simulink model "deska_ratunku"  (R2016a)
settings: Solver=VariableStepAuto  StartTime=0.0  StopTime=5000  RelTol=1e-3
values from neighbouring files (symbols this model uses):
  B = 0.0064    [Unit_3.m]    (also in reactor_pocz.m; unit_1.m; unit_4.m)
  C_lp_sg = 4314    [unit_4.m]
  c_p_PC = 5355    [Unit_3.m]    (also in unit_1.m = 5415)
  C_p_pc = 5197.6    [unit_4.m]
  c_p_PR = 6873.1    [Unit_3.m]    (also in unit_1.m)
  c_phi_1 = 2.98    [Unit_3.m]    (also in unit_1.m)
  c_phi_2 = -0.008448    [Unit_3.m]    (also in unit_1.m)
  C_psi = 13.75 * (10 ^ 6)    (= 13750000)    [Unit_3.m]    (also in reactor_pocz.m; unit_1.m; unit_4.m)
  C_vp_sg = 3449.8    [unit_4.m]
  cl_p_SG = 3809.9    [Unit_3.m]    (also in unit_1.m = 3871.3)
  cv_p_SG = 3635.6    [Unit_3.m]    (also in unit_1.m = 3489)
  E_evap_SG = 1.658 * (10 ^ 6)    (= 1658000)    [Unit_3.m]    (also in unit_1.m)
  E_evap_sg = 1.658 * (10 ^ 6)    (= 1658000)    [unit_4.m]
  K_T_SG = 9.5296 * (10 ^ 6)    (= 9529600)    [Unit_3.m]    (also in unit_1.m = 8400400)
  Kt_sg = 9.5296*(10^6)    (= 9529600)    [Unit_3.m]    (also in unit_4.m = 7554000)
  LAMBDA = 10 ^ -5    (= 1e-05)    [Unit_3.m]    (also in reactor_pocz.m; unit_1.m; unit_4.m)
  lambda = 0.1    [Unit_3.m]    (also in reactor_pocz.m; unit_1.m; unit_4.m)
  m_in = 1.4222    [Unit_3.m]    (also in unit_1.m)
  M_in = 2.19444    [unit_4.m]
  m_out = 2.11    [Unit_3.m]    (also in unit_1.m = 2.9722)
  M_out = 2.29722    [unit_4.m]
  M_PR = M_pc-V0_PC * (581.2 + 2.98*T_PC - 0.0848*(T_PC^2))    (= 1478515.60171)    [Unit_3.m]    (also in unit_1.m = 1445179.13836)
  m_SG = 119.31    [Unit_3.m]    (also in unit_1.m = 120.56)
  M_SG = 34920    [Unit_3.m]    (also in unit_1.m = 35611)
  P_1 = -1.223 * (10 ^ -4)    (= -0.0001223)    [Unit_3.m]    (also in reactor_pocz.m; unit_1.m = -0.0001322; unit_4.m = -0.0001286)
  P_2 = -5.502 * (10 ^ -5)    (= -5.502e-05)    [Unit_3.m]    (also in reactor_pocz.m; unit_1.m = -6.08e-05; unit_4.m = -6.79e-05)
  P_3 = -1.953 * (10 ^ -4)    (= -0.0001953)    [Unit_3.m]    (also in reactor_pocz.m; unit_1.m = -0.000285; unit_4.m = -0.0002887)
  S = 1938.9    [Unit_3.m]    (also in reactor_pocz.m; unit_1.m = 2859; unit_4.m = 2910.3)
  T_pc_hl = 295.21    [unit_4.m]
  T_PC_I = 258.85    [Unit_3.m]    (also in unit_1.m = 246.1)
  T_pc_i = 258.23    [unit_4.m]
  T_SG = 257.78    [Unit_3.m]    (also in unit_1.m = 255.13)
  T_SG_SW = 220.85    [Unit_3.m]    (also in unit_1.m = 219.65)
  T_sg_sw = 220.85    [unit_4.m]
  V0_PC = 242    [Unit_3.m]    (also in unit_1.m)
  V_0_pc = 242    [unit_4.m]
  W_loss_pc = 3.2733 * (10 ^ 8)    (= 327330000)    [unit_4.m]
  W_loss_PC = 2.996 * (10 ^ 7)    (= 29960000)    [Unit_3.m]    (also in unit_1.m = 224690000)
  W_loss_PR = 1.6823 * (10 ^ 5)    (= 168230)    [Unit_3.m]    (also in unit_1.m)
  W_loss_SG = 1.8932  * (10 ^ 7)    (= 18932000)    [Unit_3.m]    (also in unit_1.m = 191660)
  W_loss_sg = 1.324  * (10 ^ 7)    (= 13240000)    [unit_4.m]
libraries: simulink x2
settings Model: Creator=Użytkownik  LastModifiedBy=Użytkownik
settings GRTTargetCC: GeneratePreprocessorConditionals=Use local settings

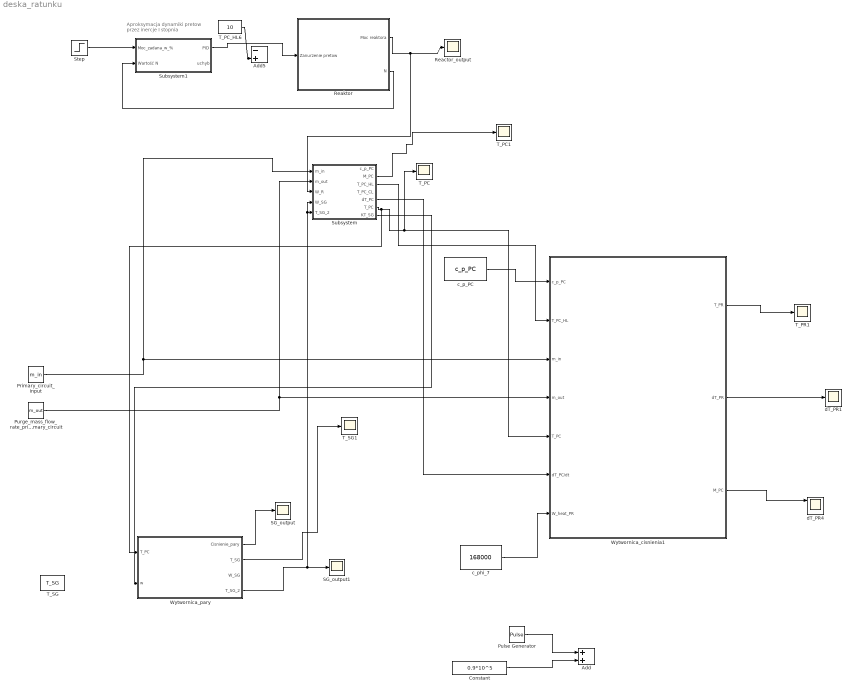
== system deska_ratunku ==
  note: Aproksymacja dynamiki
      | pretow przez inercje I stopnia
  Add : Sum
  Add5 : Sum  Inputs=-+
  Constant : Constant  Value=0.9*10^5
  Primary_circuit_input : Constant  Value=m_in
  Pulse Generator : DiscretePulseGenerator  PulseType=Time based  Amplitude=0.98*10^5  Period=6480  PulseWidth=80
  "Purge_mass_flow_rate_primary_circuit " : Constant  Value=m_out
  Reactor_output : Scope
  Reaktor : Subsystem
  SG_output : Scope
  SG_output1 : Scope
  Step : Step  Time=500  After=0.025  SampleTime=0
  Subsystem : Subsystem
  Subsystem1 : Subsystem
  T_PC : Scope
  T_PC1 : Scope
  T_PC_HL6 : Constant  Value=10
  T_PR1 : Scope
  T_SG : Constant  Value=T_SG
  T_SG1 : Scope
  Wytwornica_cisnienia1 : Subsystem
  Wytwornica_pary : Subsystem
  c_p_PC : Constant  Value=c_p_PC
  c_phi_7 : Constant  Value=168000
  dT_PR1 : Scope
  dT_PR4 : Scope  NumInputPorts=3
  wires:
  Reaktor/1(Moc reaktora) -> Subsystem/3(W_R), Reactor_output/1
  Wytwornica_pary/2(T_SG) -> T_SG1/1
  Primary_circuit_input/1 -> Subsystem/1(m_in), Wytwornica_cisnienia1/3(m_in)
  "Purge_mass_flow_rate_primary_circuit "/1 -> Subsystem/2(m_out), Wytwornica_cisnienia1/4(m_out)
  c_p_PC/1 -> Wytwornica_cisnienia1/1(c_p_PC)
  Subsystem/3(T_PC_HL) -> Wytwornica_cisnienia1/2(T_PC_HL)
  Wytwornica_cisnienia1/1(T_PR) -> T_PR1/1
  Wytwornica_cisnienia1/2(dT_PR) -> dT_PR1/1
  Pulse Generator/1 -> Add/1
  Constant/1 -> Add/2
  Subsystem/6(T_PC) -> Wytwornica_pary/1(T_PC), Wytwornica_cisnienia1/5(T_PC), T_PC/1
  Wytwornica_cisnienia1/3("M_PC ") -> dT_PR4/1
  c_phi_7/1 -> Wytwornica_cisnienia1/7(W_heat_PR)
  Subsystem/5(dT_PC) -> Wytwornica_cisnienia1/6(dT_PC/dt)
  Wytwornica_pary/1(Cisnienie_pary) -> SG_output/1
  Step/1 -> Subsystem1/1(Moc_zadana_w_%)
  Reaktor/2(N) -> Subsystem1/2(Wartość N)
  T_PC_HL6/1 -> Add5/2
  Subsystem/2(M_PC) -> T_PC1/1
  Subsystem1/1("PID ") -> Reaktor/1(Zanurzenie pretow)
  Subsystem/7("KT_SG ") -> Wytwornica_pary/2("w ")
  Wytwornica_pary/4(T_SG_2) -> Subsystem/4(W_SG), Subsystem/5(T_SG_2), SG_output1/1

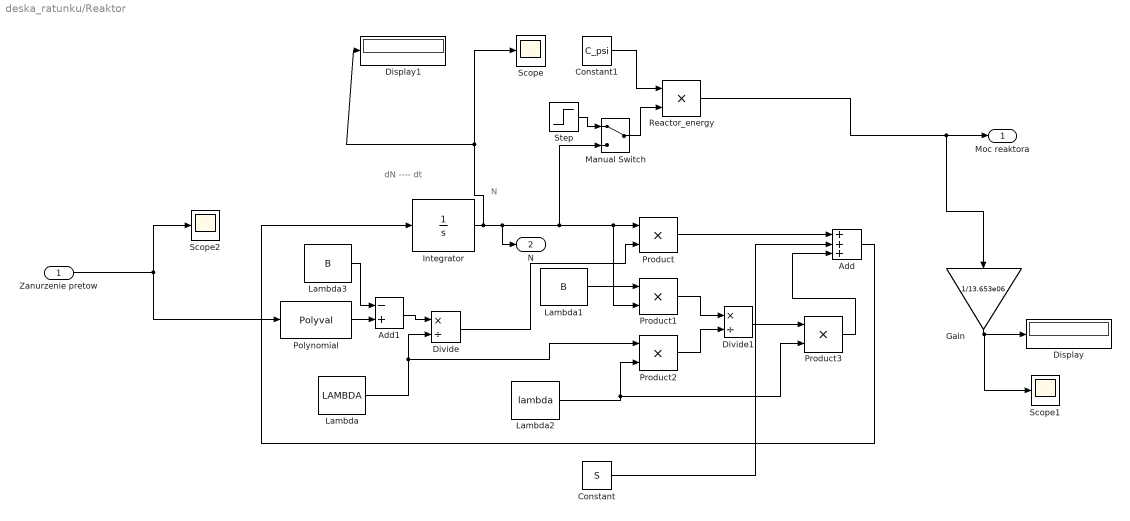
== system deska_ratunku/Reaktor ==
  note: N
  note: dN
      | ----
      | dt
  Zanurzenie pretow : Inport
  Add : Sum  Inputs=+++
  Add1 : Sum  Inputs=-+
  Constant : Constant  Value=S
  Constant1 : Constant  Value=C_psi
  Display : Display
  Display1 : Display
  Divide : Product  Inputs=*/
  Divide1 : Product  Inputs=*/
  Gain : Gain  Gain=1/13.653e06
  Integrator : Integrator  InitialCondition=99.3
  Lambda : Constant  Value=LAMBDA
  Lambda1 : Constant  Value=B
  Lambda2 : Constant  Value=lambda
  Lambda3 : Constant  Value=B
  Manual Switch : ManualSwitch
  Polynomial : Polyval  Coefs=[P_1, P_2, P_3]
  Product{,1..3} (4 alike) : Product
  Reactor_energy : Product
  Scope : Scope
  Scope1 : Scope
  Scope2 : Scope
  Step : Step  Time=500  Before=100.3  After=100.2  SampleTime=0
  Moc reaktora : Outport
  N : Outport  Port=2
  wires:
  Integrator/1 -> N/1, Manual Switch/2, Product1/2, Product/1, Display1/1, Scope/1
  Product/1 -> Add/1
  Constant/1 -> Add/2
  Add/1 -> Integrator/1
  Lambda/1 -> Product2/1, Divide/2
  Divide/1 -> Product/2
  Constant1/1 -> Reactor_energy/1
  Reactor_energy/1 -> Gain/1, Moc reaktora/1
  Lambda1/1 -> Product1/1
  Lambda2/1 -> Product2/2, Product3/2
  Product1/1 -> Divide1/1
  Product2/1 -> Divide1/2
  Divide1/1 -> Product3/1
  Product3/1 -> Add/3
  Lambda3/1 -> Add1/1
  Polynomial/1 -> Add1/2
  Add1/1 -> Divide/1
  Gain/1 -> Scope1/1, Display/1
  Zanurzenie pretow/1 -> Scope2/1, Polynomial/1
  Manual Switch/1 -> Reactor_energy/2
  Step/1 -> Manual Switch/1

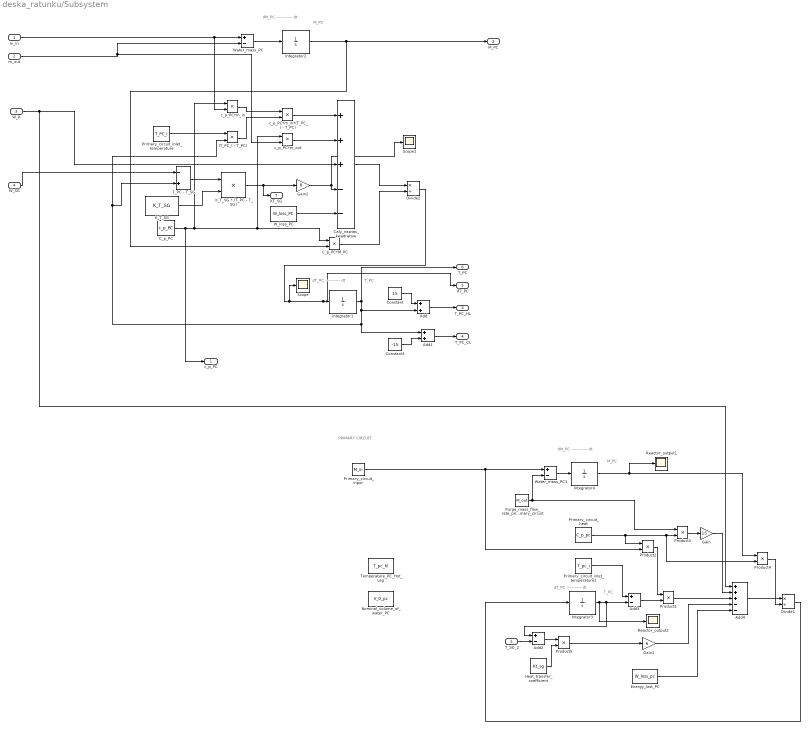
== system deska_ratunku/Subsystem ==
  note: dM_PC
      | ------------
      |      dt
  note: M_PC
  note: dT_PC
      | -----------
      |     dt
  note: T_PC
  note: dM_PC
      | ------------
      |      dt
  note: M_PC
  note: dT_PC
      | -----------
      |     dt
  note: T_PC
  note: PRIMARY CIRCUIT
  m_in : Inport
  m_out : Inport  Port=2
  W_R : Inport  Port=3
  W_SG : Inport  Port=4
  T_SG_2 : Inport  Port=5
  (T_PC_I - T_PC) : Product
  Add : Sum
  Add1 : Sum
  Add2 : Sum  Inputs=+-
  Add3 : Sum  Inputs=+-
  Add4 : Sum  Inputs=+++--
  C_p_PC : Constant  Value=c_p_PC
  C_p_PC*M_PC : Product
  Caly_nawias_kwadratow : Sum  Inputs=+++--
  Constant : Constant  Value=15
  Constant1 : Constant  Value=-15
  Divide1 : Product  Inputs=*/
  Divide2 : Product  Inputs=*/
  Energy_lost_PC : Constant  Value=W_loss_pc
  Gain : Gain  Gain=15
  Gain1 : Gain  Gain=6
  Gain2 : Gain  Gain=6
  Heat_transfer_coefficient : Constant  Value=Kt_sg
  Integrator1 : Integrator  InitialCondition=281.13
  Integrator2 : Integrator  InitialCondition=200000
  Integrator3 : Integrator  InitialCondition=281.13
  Integrator4 : Integrator  InitialCondition=200000
  K_T_SG : Constant  Value=K_T_SG
  K_T_SG * (T_PC - T_SG) : Product
  Nominal_volume_of_water_PC : Constant  Value=V_0_pc
  Primary_circuit_heat : Constant  Value=C_p_pc
  Primary_circuit_inlet_temperature : Constant  Value=T_PC_I
  Primary_circuit_inlet_temperature1 : Constant  Value=T_pc_i
  Primary_circuit_input : Constant  Value=M_in
  Product{1..5} (5 alike) : Product
  "Purge_mass_flow_rate_primary_circuit " : Constant  Value=M_out
  Reactor_output1 : Scope
  Reactor_output2 : Scope
  Scope : Scope
  Scope1 : Scope
  T_PC - T_SG : Sum  Inputs=-+
  Temperature_PC_Hot_Leg : Constant  Value=T_pc_hl
  W_loss_PC : Constant  Value=W_loss_PC
  Water_mass_PC : Sum  Inputs=+-
  Water_mass_PC1 : Sum  Inputs=+-
  c_p_PC*m_in : Product
  c_p_PC*m_in*(T_PC_I - T_PC) : Product
  c_p_PC*m_out : Product
  c_p_PC : Outport
  M_PC : Outport  Port=2
  T_PC_HL : Outport  Port=3
  T_PC_CL : Outport  Port=4
  dT_PC : Outport  Port=5
  T_PC : Outport  Port=6
  "KT_SG " : Outport  Port=7
  wires:
  m_in/1 -> c_p_PC*m_in/2, Water_mass_PC/1
  Water_mass_PC/1 -> Integrator2/1
  Integrator2/1 -> C_p_PC*M_PC/2, M_PC/1
  C_p_PC/1 -> c_p_PC/1, C_p_PC*M_PC/1, c_p_PC*m_out/1, c_p_PC*m_in/1
  C_p_PC*M_PC/1 -> Divide2/2
  Divide2/1 -> Scope/1, dT_PC/1, Integrator1/1
  Caly_nawias_kwadratow/1 -> Divide2/1
  c_p_PC*m_in*(T_PC_I - T_PC)/1 -> Caly_nawias_kwadratow/1
  c_p_PC*m_in/1 -> c_p_PC*m_in*(T_PC_I - T_PC)/1
  (T_PC_I - T_PC)/1 -> c_p_PC*m_in*(T_PC_I - T_PC)/2
  Primary_circuit_inlet_temperature/1 -> (T_PC_I - T_PC)/1
  c_p_PC*m_out/1 -> Caly_nawias_kwadratow/2
  W_loss_PC/1 -> Caly_nawias_kwadratow/5
  Constant/1 -> Add/1
  Constant1/1 -> Add1/2
  Integrator1/1 -> T_PC - T_SG/2, (T_PC_I - T_PC)/2, Add1/1, Add/2, T_PC/1
  Add1/1 -> T_PC_CL/1
  Add/1 -> T_PC_HL/1
  m_out/1 -> c_p_PC*m_out/2, Water_mass_PC/2
  Gain2/1 -> Caly_nawias_kwadratow/4, Scope1/1
  T_PC - T_SG/1 -> K_T_SG * (T_PC - T_SG)/1
  K_T_SG/1 -> K_T_SG * (T_PC - T_SG)/2
  K_T_SG * (T_PC - T_SG)/1 -> "KT_SG "/1, Gain2/1
  W_SG/1 -> T_PC - T_SG/1
  W_R/1 -> Add4/1, Caly_nawias_kwadratow/3
  Primary_circuit_input/1 -> Water_mass_PC1/1, Product2/2
  "Purge_mass_flow_rate_primary_circuit "/1 -> Water_mass_PC1/2, Product3/1
  Water_mass_PC1/1 -> Integrator4/1
  Integrator3/1 -> Reactor_output2/1, Add2/1, Add3/2
  Primary_circuit_inlet_temperature1/1 -> Add3/1
  Add3/1 -> Product1/2
  Product2/1 -> Product1/1
  Primary_circuit_heat/1 -> Product2/1, Product4/2, Product3/2
  Product1/1 -> Add4/3
  Product3/1 -> Gain/1
  Gain/1 -> Add4/2
  Product5/1 -> Gain1/1
  Gain1/1 -> Add4/4
  Add4/1 -> Divide1/1
  Integrator4/1 -> Reactor_output1/1, Product4/1
  Product4/1 -> Divide1/2
  Divide1/1 -> Integrator3/1
  Heat_transfer_coefficient/1 -> Product5/2
  Add2/1 -> Product5/1
  Energy_lost_PC/1 -> Add4/5
  T_SG_2/1 -> Add2/2

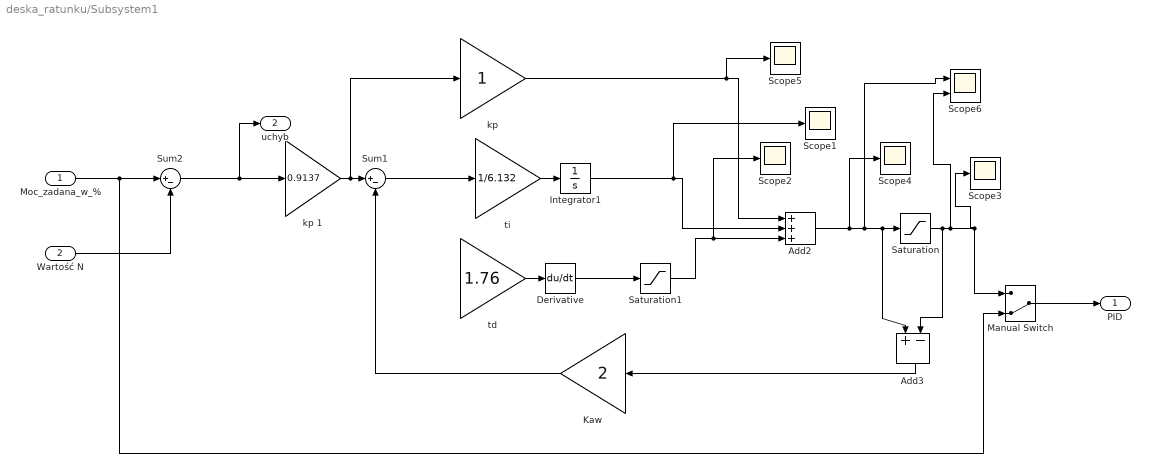
== system deska_ratunku/Subsystem1 ==
  Moc_zadana_w_% : Inport
  Wartość N : Inport  Port=2
  " kp " : Gain
  " kp 1" : Gain  Gain=0.9137
  Add2 : Sum  Inputs=+++
  Add3 : Sum  Inputs=+-
  Derivative : Derivative
  Integrator1 : Integrator
  "Kaw " : Gain  Gain=2
  Manual Switch : ManualSwitch  CurrentSetting=0
  Saturation : Saturate  UpperLimit=10  LowerLimit=0
  Saturation1 : Saturate  UpperLimit=10  LowerLimit=-10
  Scope{1..5} (5 alike) : Scope
  Scope6 : Scope  NumInputPorts=2
  Sum1 : Sum  Inputs=|+-
  Sum2 : Sum  Inputs=|+-
  "td " : Gain  Gain=1.76
  ti : Gain  Gain=1/6.132
  "PID " : Outport
  uchyb : Outport  Port=2
  wires:
  Derivative/1 -> Saturation1/1
  Add2/1 -> Scope6/1, Add3/1, Saturation/1, Scope4/1
  Saturation/1 -> Add3/2, Scope6/2, Scope3/1, Manual Switch/1
  Wartość N/1 -> Sum2/2
  Manual Switch/1 -> "PID "/1
  Moc_zadana_w_%/1 -> Manual Switch/2, Sum2/1
  ti/1 -> Integrator1/1
  "td "/1 -> Derivative/1
  Add3/1 -> "Kaw "/1
  " kp 1"/1 -> " kp "/1, Sum1/1
  Sum1/1 -> ti/1
  Saturation1/1 -> Scope2/1, Add2/3
  Integrator1/1 -> Scope1/1, Add2/2
  " kp "/1 -> Scope5/1, Add2/1
  Sum2/1 -> uchyb/1, " kp 1"/1
  "Kaw "/1 -> Sum1/2

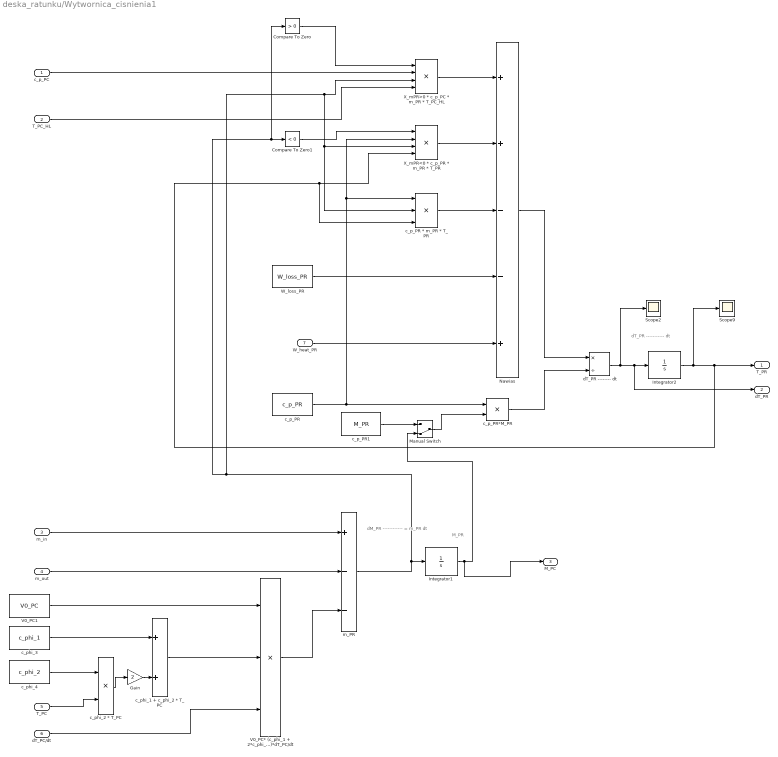
== system deska_ratunku/Wytwornica_cisnienia1 ==
  note: dT_PR
      | -----------
      | dt
  note: dM_PR
      | ------------ = m_PR
      |     dt
  note: M_PR
  c_p_PC : Inport
  T_PC_HL : Inport  Port=2
  m_in : Inport  Port=3
  m_out : Inport  Port=4
  T_PC : Inport  Port=5
  dT_PC/dt : Inport  Port=6
  W_heat_PR : Inport  Port=7
  Compare To Zero : simulink/Logic and Bit Operations/Compare To Zero  relop=>  OutDataTypeStr=boolean
  Compare To Zero1 : simulink/Logic and Bit Operations/Compare To Zero  relop=<  OutDataTypeStr=boolean
  Gain : Gain  Gain=2
  Integrator1 : Integrator  InitialCondition=19400
  Integrator2 : Integrator  InitialCondition=326.57
  Manual Switch : ManualSwitch  CurrentSetting=0
  Nawias : Sum  Inputs=++--+
  Scope2 : Scope
  Scope9 : Scope
  V0_PC* (c_phi_1 + 2*c_phi_2*T_PC)*dT_PC/dt : Product  Inputs=3
  V0_PC1 : Constant  Value=V0_PC
  W_loss_PR : Constant  Value=W_loss_PR
  X_mPR<0 * c_p_PR * m_PR * T_PR : Product  Inputs=4
  X_mPR>0 * c_p_PC * m_PR * T_PC_HL : Product  Inputs=4
  c_p_PR : Constant  Value=c_p_PR
  c_p_PR * m_PR * T_PR : Product  Inputs=3
  c_p_PR*M_PR : Product
  c_p_PR1 : Constant  Value=M_PR
  "c_phi_1 + c_phi_2 * T_PC " : Sum
  c_phi_2 * T_PC : Product
  c_phi_3 : Constant  Value=c_phi_1
  c_phi_4 : Constant  Value=c_phi_2
  dT_PR -------- dt : Product  Inputs=*/
  m_PR : Sum  Inputs=+--
  T_PR : Outport
  dT_PR : Outport  Port=2
  "M_PC " : Outport  Port=3
  wires:
  c_p_PR*M_PR/1 -> dT_PR -------- dt/2
  Nawias/1 -> dT_PR -------- dt/1
  c_p_PR/1 -> X_mPR<0 * c_p_PR * m_PR * T_PR/2, c_p_PR * m_PR * T_PR/1, c_p_PR*M_PR/1
  Compare To Zero/1 -> X_mPR>0 * c_p_PC * m_PR * T_PC_HL/1
  X_mPR>0 * c_p_PC * m_PR * T_PC_HL/1 -> Nawias/1
  c_p_PC/1 -> X_mPR>0 * c_p_PC * m_PR * T_PC_HL/2
  m_PR/1 -> Compare To Zero/1, Compare To Zero1/1, X_mPR>0 * c_p_PC * m_PR * T_PC_HL/3, c_p_PR * m_PR * T_PR/2, X_mPR<0 * c_p_PR * m_PR * T_PR/3, Integrator1/1
  T_PC_HL/1 -> X_mPR>0 * c_p_PC * m_PR * T_PC_HL/4
  X_mPR<0 * c_p_PR * m_PR * T_PR/1 -> Nawias/2
  Compare To Zero1/1 -> X_mPR<0 * c_p_PR * m_PR * T_PR/1
  Integrator2/1 -> Scope9/1, X_mPR<0 * c_p_PR * m_PR * T_PR/4, c_p_PR * m_PR * T_PR/3, T_PR/1
  c_p_PR * m_PR * T_PR/1 -> Nawias/3
  W_heat_PR/1 -> Nawias/5
  W_loss_PR/1 -> Nawias/4
  m_in/1 -> m_PR/1
  m_out/1 -> m_PR/2
  V0_PC* (c_phi_1 + 2*c_phi_2*T_PC)*dT_PC/dt/1 -> m_PR/3
  V0_PC1/1 -> V0_PC* (c_phi_1 + 2*c_phi_2*T_PC)*dT_PC/dt/1
  "c_phi_1 + c_phi_2 * T_PC "/1 -> V0_PC* (c_phi_1 + 2*c_phi_2*T_PC)*dT_PC/dt/2
  c_phi_3/1 -> "c_phi_1 + c_phi_2 * T_PC "/1
  c_phi_2 * T_PC/1 -> Gain/1
  Gain/1 -> "c_phi_1 + c_phi_2 * T_PC "/2
  c_phi_4/1 -> c_phi_2 * T_PC/1
  T_PC/1 -> c_phi_2 * T_PC/2
  dT_PR -------- dt/1 -> Scope2/1, dT_PR/1, Integrator2/1
  dT_PC/dt/1 -> V0_PC* (c_phi_1 + 2*c_phi_2*T_PC)*dT_PC/dt/3
  Integrator1/1 -> "M_PC "/1, Manual Switch/2
  c_p_PR1/1 -> Manual Switch/1
  Manual Switch/1 -> c_p_PR*M_PR/2

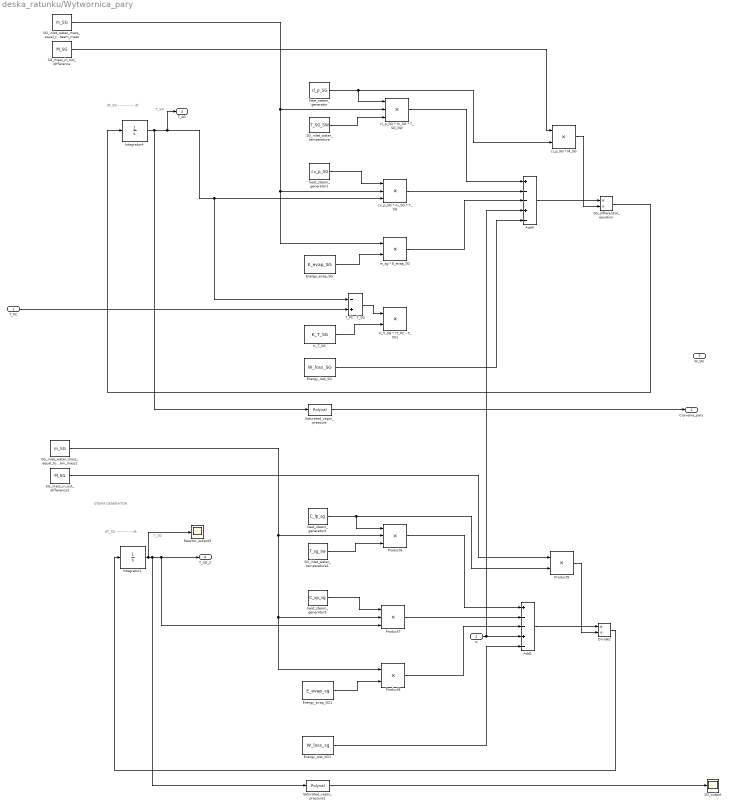
== system deska_ratunku/Wytwornica_pary ==
  note: T_SG
  note: dT_SG
      | ------------
      |     dt
  note: T_SG
  note: dT_SG
      | ------------
      |     dt
  note: STEAM GENERATOR
  T_PC : Inport
  "w " : Inport  Port=2
  Add1 : Sum  Inputs=+--+-
  Add4 : Sum  Inputs=+--+-
  Divide2 : Product  Inputs=*/
  Energy_evap_SG : Constant  Value=E_evap_SG
  Energy_evap_SG1 : Constant  Value=E_evap_sg
  Energy_lost_SG : Constant  Value=W_loss_SG
  Energy_lost_SG1 : Constant  Value=W_loss_sg
  Integrator1 : Integrator  InitialCondition=257.78
  Integrator4 : Integrator  InitialCondition=257.78
  K_T_SG : Constant  Value=K_T_SG
  K_T_SG * (T_PC - T_SG) : Product
  Product6 : Product  Inputs=3
  Product7 : Product  Inputs=3
  Product8 : Product
  Product9 : Product
  Reactor_output3 : Scope
  SG_differential_equation : Product  Inputs=*/
  SG_inlet_water_mass_equal_to_outlet_steam_mass : Constant  Value=m_SG
  SG_inlet_water_mass_equal_to_outlet_steam_mass1 : Constant  Value=m_SG
  SG_inlet_water_temperature : Constant  Value=T_SG_SW
  SG_inlet_water_temperature1 : Constant  Value=T_sg_sw
  SG_mass_in_out_difference : Constant  Value=M_SG
  SG_mass_in_out_difference1 : Constant  Value=M_SG
  SG_output : Scope
  Saturated_vapor_pressure : Polyval  Coefs=[0.63, -258.01, 28884.78]
  Saturated_vapor_pressure1 : Polyval  Coefs=[0.63, -258.01, 28884.78]
  T_PC - T_SG : Sum  Inputs=-+
  cl_p_SG * M_SG : Product
  cl_p_SG * m_SG * T_SG_SW : Product  Inputs=3
  cv_p_SG * m_SG * T_SG : Product  Inputs=3
  heat_steam_generator : Constant  Value=cl_p_SG
  heat_steam_generator1 : Constant  Value=cv_p_SG
  heat_steam_generator2 : Constant  Value=C_lp_sg
  heat_steam_generator3 : Constant  Value=C_vp_sg
  m_sg * E_evap_SG : Product
  Cisnienie_pary : Outport
  T_SG : Outport  Port=2
  "W_SG " : Outport  Port=3
  T_SG_2 : Outport  Port=4
  wires:
  heat_steam_generator/1 -> cl_p_SG * M_SG/2, cl_p_SG * m_SG * T_SG_SW/1
  SG_inlet_water_mass_equal_to_outlet_steam_mass/1 -> m_sg * E_evap_SG/1, cv_p_SG * m_SG * T_SG/2, cl_p_SG * m_SG * T_SG_SW/2
  SG_inlet_water_temperature/1 -> cl_p_SG * m_SG * T_SG_SW/3
  heat_steam_generator1/1 -> cv_p_SG * m_SG * T_SG/1
  Integrator4/1 -> Saturated_vapor_pressure/1, T_SG/1, T_PC - T_SG/1, cv_p_SG * m_SG * T_SG/3
  Energy_evap_SG/1 -> m_sg * E_evap_SG/2
  cl_p_SG * m_SG * T_SG_SW/1 -> Add4/1
  cv_p_SG * m_SG * T_SG/1 -> Add4/2
  m_sg * E_evap_SG/1 -> Add4/3
  Energy_lost_SG/1 -> Add4/5
  Add4/1 -> SG_differential_equation/1
  SG_mass_in_out_difference/1 -> cl_p_SG * M_SG/1
  cl_p_SG * M_SG/1 -> SG_differential_equation/2
  SG_differential_equation/1 -> Integrator4/1
  Saturated_vapor_pressure/1 -> Cisnienie_pary/1
  T_PC - T_SG/1 -> K_T_SG * (T_PC - T_SG)/1
  T_PC/1 -> T_PC - T_SG/2
  K_T_SG/1 -> K_T_SG * (T_PC - T_SG)/2
  heat_steam_generator2/1 -> Product9/2, Product6/1
  SG_inlet_water_mass_equal_to_outlet_steam_mass1/1 -> Product8/1, Product7/2, Product6/2
  SG_inlet_water_temperature1/1 -> Product6/3
  heat_steam_generator3/1 -> Product7/1
  Integrator1/1 -> Reactor_output3/1, Saturated_vapor_pressure1/1, T_SG_2/1, Product7/3
  Energy_evap_SG1/1 -> Product8/2
  Product6/1 -> Add1/1
  Product7/1 -> Add1/2
  Product8/1 -> Add1/3
  Energy_lost_SG1/1 -> Add1/5
  Add1/1 -> Divide2/1
  SG_mass_in_out_difference1/1 -> Product9/1
  Product9/1 -> Divide2/2
  Divide2/1 -> Integrator1/1
  Saturated_vapor_pressure1/1 -> SG_output/1
  "w "/1 -> Add4/4, Add1/4
